simulink model "attitude_loop"  (R2016a)
settings: Solver=VariableStepAuto  StartTime=0.0  StopTime=10  RelTol=1e-3
values from neighbouring files (symbols this model uses):
  g = 9.81    [controller_script.m]
  I = [0.06 0.003 0.0006;0.003 0.05 0.002;0.002 0.003 0.1]    [controller_script.m]
  Kr = 20*eye(3)    [controller_script.m]
  Kw = 2*eye(3)    [controller_script.m]
  m = 1.5    [controller_script.m]
  zw = [0;0;1]    [controller_script.m]
settings Model: Creator=hugoa  LastModifiedBy=hugoa

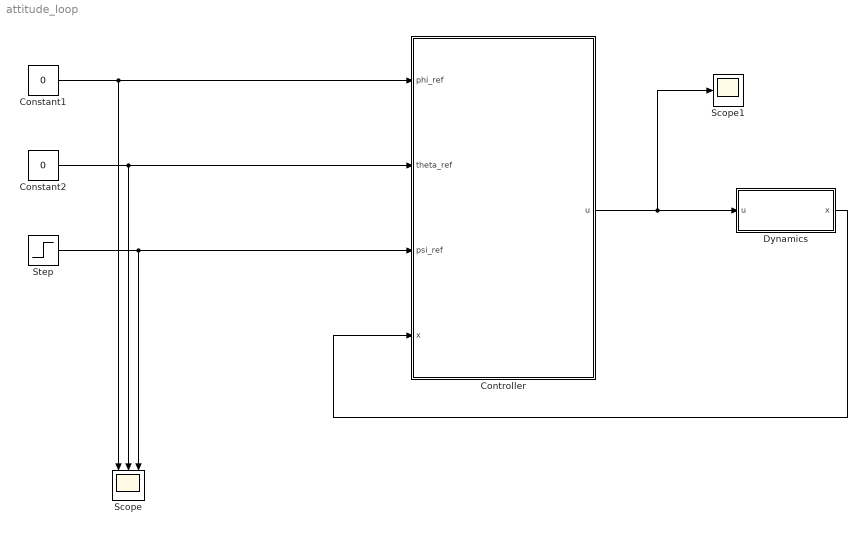
== system attitude_loop ==
  Constant1 : Constant  Value=0
  Constant2 : Constant  Value=0
  "Controller " : Subsystem
  Dynamics : Subsystem
  Scope : Scope  NumInputPorts=3
  Scope1 : Scope
  Step : Step  After=pi  SampleTime=0
  wires:
  Dynamics/1(x) -> "Controller "/4(x)
  "Controller "/1(u) -> Scope1/1, Dynamics/1(u)
  Constant1/1 -> "Controller "/1(phi_ref), Scope/1
  Step/1 -> "Controller "/3(psi_ref), Scope/3
  Constant2/1 -> "Controller "/2(theta_ref), Scope/2

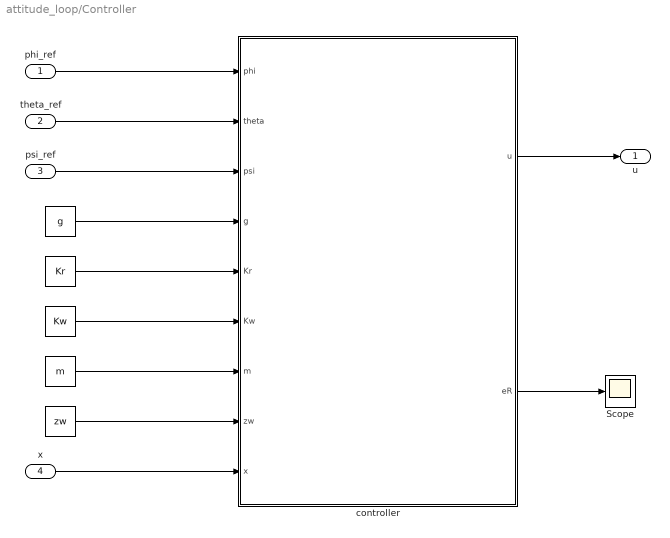
== system attitude_loop/Controller  ==
  phi_ref : Inport
  theta_ref : Inport  Port=2
  psi_ref : Inport  Port=3
  x : Inport  Port=4
  " " : Constant  Value=g
  "  " : Constant  Value=Kr
  "   " : Constant  Value=Kw
  "     " : Constant  Value=m
  "      " : Constant  Value=zw
  Scope : Scope
  controller : MATLAB Function  TreatAsAtomicUnit=on
  u : Outport
  wires:
  " "/1 -> controller/4(g)
  controller/1(u) -> u/1
  "  "/1 -> controller/5(Kr)
  "   "/1 -> controller/6(Kw)
  "      "/1 -> controller/8(zw)
  "     "/1 -> controller/7(m)
  x/1 -> controller/9(x)
  psi_ref/1 -> controller/3(psi)
  theta_ref/1 -> controller/2(theta)
  phi_ref/1 -> controller/1(phi)
  controller/2(eR) -> Scope/1

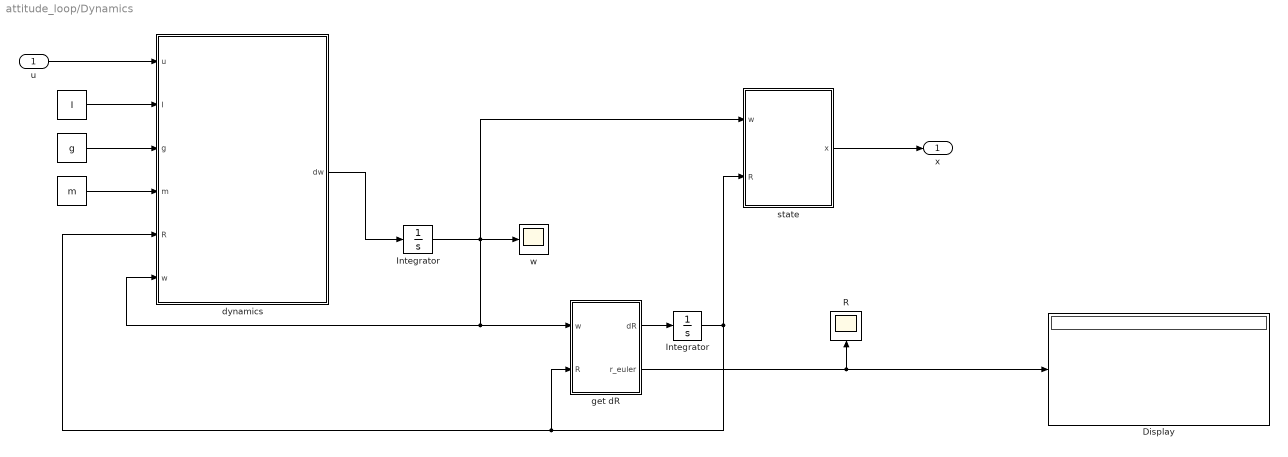
== system attitude_loop/Dynamics ==
  u : Inport
  " " : Constant  Value=I
  "  " : Constant  Value=g
  "   " : Constant  Value=m
  Display : Display
  "Integrator " : Integrator  InitialCondition=eye(3)  LimitOutput=on  UpperSaturationLimit=1  LowerSaturationLimit=0
  "Integrator " : Integrator  InitialCondition=[0;0;0]
  R : Scope
  dynamics : MATLAB Function  TreatAsAtomicUnit=on
  get dR : MATLAB Function  TreatAsAtomicUnit=on
  state : MATLAB Function  TreatAsAtomicUnit=on
  w : Scope
  x : Outport
  wires:
  "Integrator "/1 -> state/1(w), w/1, dynamics/6(w), get dR/1(w)
  "Integrator "/1 -> dynamics/5(R), get dR/2(R), state/2(R)
  state/1(x) -> x/1
  " "/1 -> dynamics/2(I)
  get dR/1(dR) -> "Integrator "/1
  "   "/1 -> dynamics/4(m)
  "  "/1 -> dynamics/3(g)
  u/1 -> dynamics/1(u)
  get dR/2(r_euler) -> R/1, Display/1
  dynamics/1(dw) -> "Integrator "/1

== matlab function attitude_loop/Dynamics/get dR ==
  data: dR output; w input; R input; r_euler output
function [dR, r_euler] = fcn(w, R)
%#codegen
skew_w = [0,-w(3),w(2); w(3),0,-w(1); -w(2),w(1),0];



dR = R*skew_w;
r_euler = rotm2eul(R);

== matlab function attitude_loop/Dynamics/dynamics ==
  data: u input; I input; g input; m input; R input; dw output; w input size=3
function dw = fcn(u,I,g,m,R,w)
%#codegen
zw = [0;0;1];
zB = R*zw;

skew_w = [0,-w(3),w(2); w(3),0,-w(1); -w(2),w(1),0];
uT = [u(2);u(3);u(4)];



%dw = inv(I)*(-skew_w*I*w + uT);
dw = inv(I)*((cross(-w,I*w))+uT);

== matlab function attitude_loop/Dynamics/state ==
  data: w input; R input; x output
function x = fcn(w, R)
%#codegen

x = [w, R];

== matlab function attitude_loop/Controller /controller ==
  data: phi input; theta input; psi input; g input; Kr input; Kw input; m input; zw input; u output; x input; eR output
function [u,eR]    = fcn(phi, theta, psi,g, Kr, Kw, m, zw, x)

%% CONSTANTS
    Kp = [15,0,0; 0,15,0; 0,0,15];
    Kv = [10,0,0; 0,10,0; 0,0,10];
%%%%%%%%%%%%%%%%%%%%%%%%%%%%%%%%%%%%%%%%%%%%%%%

%% REFERENCE INPUT -> TO BE CHANGED 
    %Position reference
    p_ref = [0;0;0];
    %Velocity reference
    v_ref = [0;0;0];
    %Angular velocity reference
    %wb_ref = [0;0;0];
    %Acceleration reference
    a_ref = [0;0;0];
    %Phi angle reference
    psi_ref = 0;
    % Jerk reference
    jerk = [0;0;0];
    R_des = [cos(psi)*cos(theta)-sin(phi)*sin(psi)*sin(theta) -cos(phi)*sin(psi) cos(psi)*sin(theta)+cos(theta)*sin(phi)*sin(psi);...
        cos(theta)*sin(psi)+cos(psi)*sin(phi)*sin(theta) cos(phi)*cos(psi) sin(psi)*sin(theta)-cos(psi)*cos(theta)*sin(phi);...
        -cos(phi)*sin(theta) sin(phi) cos(phi)*cos(theta)];
    

%%%%%%%%%%%%%%%%%%%%%%%%%%%%%%%%%%%%%%%%%%%%%%%

%% GET THE STATE
    wb = x(1:3,1);
    %Rotation matrix
    R = x(1:3,2:4);
%%%%%%%%%%%%%%%%%%%%%%%%%%%%%%%%%%%%%%%%%%%%%%%

%% EQUATIONS
   
    zB = R*zw;
    % COMO CALCULO U1 AQUI????????????'
    F_des = [0;0;0];
    u1= dot(F_des, zB);
    
    %Orientation Error
    eR_aux = (transpose(R_des)*R - transpose(R)*R_des);
    eR = 0.5 * [eR_aux(3,2); eR_aux(1,3); eR_aux(2,1)];

    %Angular velocity
    h = m/u1*(jerk - ( dot(zB_des, jerk)*zB_des));
    p_des = dot(-h,yB_des);
    q_des = dot(h,xB_des);
    % VERY BAD
    r_des = 0;
    wb_ref = [p_des; q_des; r_des];
    
    %Angular Velocity Error
    ew = wb - wb_ref; 

    
%%%%%%%%%%%%%%%%%%%%%%%%%%%%%%%%%%%%%%%%%%%%%%%

%% OUTPUT

    uT = - Kr*eR - Kw*ew;
    u = [u1; uT];
 
%%%%%%%%%%%%%%%%%%%%%%%%%%%%%%%%%%%%%%%%%%%%%%%
